simulink model "bpskdemo"  (Simulink 4.00)
settings: Solver=ode45  StartTime=0.0  StopTime=999999  FixedStep=.0001  MaxStep=.0001  MinStep=.00000001  RelTol=1e-3  AbsTol=1e-3
settings Model: Creator=gerhard  BlockReductionOpt=off

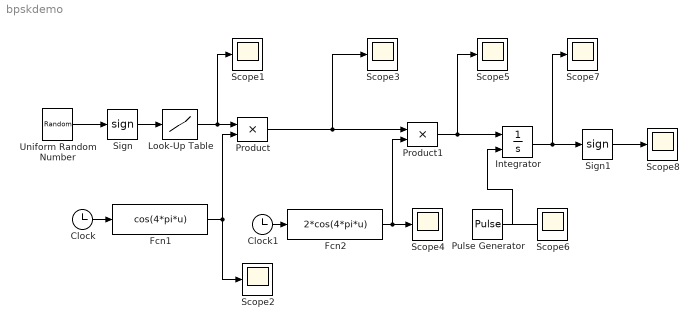
== system bpskdemo ==
  Clock : Clock
      settings: DisplayTime=off  Decimation=10
  Clock1 : Clock
      settings: DisplayTime=off  Decimation=10
  Fcn1 : Fcn  Expr=cos(4*pi*u)
  Fcn2 : Fcn  Expr=2*cos(4*pi*u)
  Integrator : Integrator  ExternalReset=rising  InitialConditionSource=internal  InitialCondition=0  LimitOutput=off  UpperSaturationLimit=inf  LowerSaturationLimit=-inf  ShowSaturationPort=off  ShowStatePort=off  AbsoluteTolerance=auto
  Look-Up Table : Lookup  InputValues=[-1,0,1]  OutputValues=[-1,1,1]
  Product : Product  Inputs=2  Multiplication=Element-wise(.*)  SaturateOnIntegerOverflow=on
  Product1 : Product  Inputs=2  Multiplication=Element-wise(.*)  SaturateOnIntegerOverflow=on
  Pulse Generator : DiscretePulseGenerator  PulseType=Time-based  Amplitude=1  Period=1  PulseWidth=50  PhaseDelay=0  SampleTime=1
  Scope{1..8} (8 alike) : Scope
      Scope1 settings: TimeRange=10  YMin=-5  YMax=5  SaveToWorkspace=off  SaveName=ScopeData3  LimitDataPoints=on  MaxDataPoints=5000
      Scope2 settings: TimeRange=10  YMin=-5  YMax=5  SaveToWorkspace=off  SaveName=ScopeData  LimitDataPoints=on  MaxDataPoints=5000
      Scope3 settings: TimeRange=10  YMin=-5  YMax=5  SaveToWorkspace=off  LimitDataPoints=on  MaxDataPoints=5000
      Scope4 settings: TimeRange=10  YMin=-5  YMax=5  SaveToWorkspace=off  SaveName=ScopeData5  LimitDataPoints=on  MaxDataPoints=5000
      Scope5 settings: TimeRange=10  YMin=-5  YMax=5  SaveToWorkspace=off  SaveName=ScopeData4  LimitDataPoints=on  MaxDataPoints=5000
      Scope6 settings: TimeRange=10  YMin=-5  YMax=5  SaveToWorkspace=off  SaveName=ScopeData7  LimitDataPoints=on  MaxDataPoints=5000
      Scope7 settings: TimeRange=10  YMin=-5  YMax=5  SaveToWorkspace=off  SaveName=ScopeData6  LimitDataPoints=on  MaxDataPoints=5000
      Scope8 settings: TimeRange=10  YMin=-5  YMax=5  SaveToWorkspace=off  SaveName=ScopeData2  LimitDataPoints=on  MaxDataPoints=5000
  Sign : Signum
  Sign1 : Signum
  Uniform Random Number : UniformRandomNumber  Minimum=-1  Maximum=1  Seed=0  SampleTime=1
  wires:
  Clock/1 -> Fcn1/1
  Fcn1/1 -> Product/2, Scope2/1
  Clock1/1 -> Fcn2/1
  Fcn2/1 -> Scope4/1, Product1/2
  Product1/1 -> Scope5/1, Integrator/1
  Integrator/1 -> Scope7/1, Sign1/1
  Pulse Generator/1 -> Integrator/2, Scope6/1
  Product/1 -> Scope3/1, Product1/1
  Sign1/1 -> Scope8/1
  Uniform Random Number/1 -> Sign/1
  Sign/1 -> Look-Up Table/1
  Look-Up Table/1 -> Product/1, Scope1/1
